simulink model "simulation"  (R2020a)
settings: Solver=ode4  StartTime=0.0  StopTime=10.0  FixedStep=dt  RelTol=1e-3
values from neighbouring files (symbols this model uses):
  alt0 = 600    [initializeSim.m]
  dt = 0.1    [dryden_wind_model.m]    (also in filters.m; full_sim_and_filter_loop.m = 0.01; getDynamicsJacobian.m; initializeSim.m = 0.01)
  F = [0;0;0]    [simple_sim.m]
  initCovarianceEkf = diag([1e-3, 1e-3,                            2, 5e-3,                            1e-4, 1e-4,                            10, 10])    [initializeSim.m]
  initEstimateEkf = [0, 0,                     initGroundSpeedEst, initAttitude(3),                     windNorthStatic + 4*randn, windEastStatic + 4*randn,                     0, 0]    [initializeSim.m]
  q = uKF(2)    [dynJacobian.m]    (also in getDynamicsJacobian.m; getDynamicsJacobianTest.m; getStateTransitionDynamics.m; simple_sim.m)
  Qekf = diag([1e-5, 1e-5,               1, 1e-3,               1, 1,               1, 1])    [initializeSim.m]
  r = uKF(3)    [dynJacobian.m]    (also in getDynamicsJacobian.m; getDynamicsJacobianTest.m; getStateTransitionDynamics.m; simple_sim.m)
  Rekf = diag([1, 1,               1, 1e-3,               1, 1])    [initializeSim.m]
  sensorNoiseFlag = 1    [initializeSim.m]
  staticWindFlag = 1    [initializeSim.m]
  turbulentWindFlag = 1    [initializeSim.m]
  windDownStatic = 0    [initializeSim.m]
  windEastStatic = -9    [initializeSim.m]
  windNorthStatic = 14    [initializeSim.m]
undefined symbols (not defined in the file or in its folder): Light, MIL
libraries: shared6dof x1, aerolibwind2 x1
settings Model: Creator=Don  LastModifiedBy=don

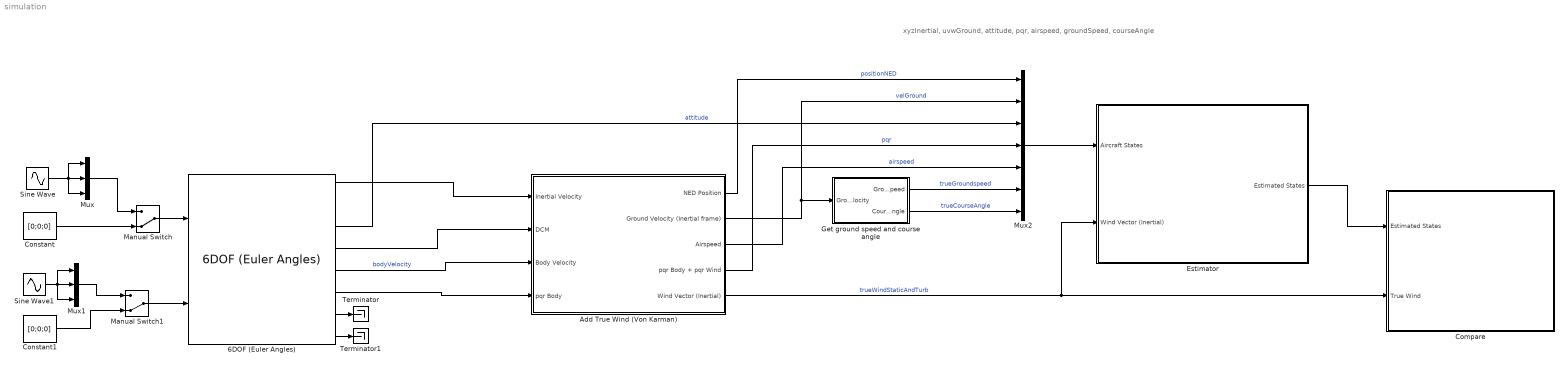
== system simulation ==
  note: xyzInertial, uvwGround, attitude, pqr, airspeed, groundSpeed, courseAngle
  6DOF (Euler Angles) : shared6dof/6DOF (Euler Angles)  units=Metric (MKS)  mtype=Fixed  rep=Euler Angles  xme_0=[0 0 -abs(alt0)]  Vm_0=initVelBody  eul_0=initAttitude  pm_0=[0 0 0]  mass_0=mass  mass_e=0.5  mass_f=2.0  inertia=J  inertia_e=eye(3)  inertia_f=2*eye(3)  k_quat=1.0  vre_flag=on  abi_flag=off  aMode=0  xme_statename=''  Vm_statename=''  eul_statename=''  quat_statename=''  pm_statename=''  mass_statename=''
      settings: SourceProductBaseCode=AE,PW,MT,VE,VP
  Add True Wind (Von Karman) : Subsystem
  Compare : Subsystem
  Constant : Constant  Value=[0;0;0]
  Constant1 : Constant  Value=[0;0;0]
  Estimator : Subsystem
  Get ground speed and course angle : Subsystem
  Manual Switch : ManualSwitch  CurrentSetting=0
  Manual Switch1 : ManualSwitch  CurrentSetting=0
  Mux : Mux  Inputs=3
  Mux1 : Mux  Inputs=3
  Mux2 : Mux  Inputs=7
  Sine Wave : Sin  SampleTime=0
  Sine Wave1 : Sin  SampleTime=0
  Terminator : Terminator
  Terminator1 : Terminator
  wires:
  Constant/1 -> Manual Switch/2
  Constant1/1 -> Manual Switch1/2
  6DOF (Euler Angles)/1 -> Add True Wind (Von Karman)/1(Inertial Velocity)
  6DOF (Euler Angles)/4 -> Add True Wind (Von Karman)/2(DCM)
  6DOF (Euler Angles)/5 -> Add True Wind (Von Karman)/3(Body Velocity)  "bodyVelocity"
  6DOF (Euler Angles)/6 -> Add True Wind (Von Karman)/4(pqr Body)
  Manual Switch/1 -> 6DOF (Euler Angles)/1
  Manual Switch1/1 -> 6DOF (Euler Angles)/2
  Sine Wave/1 -> Mux/2, Mux/1, Mux/3
  Mux/1 -> Manual Switch/1
  Sine Wave1/1 -> Mux1/2, Mux1/1, Mux1/3
  Mux1/1 -> Manual Switch1/1
  Add True Wind (Von Karman)/2(Ground Velocity (Inertial frame)) -> Mux2/2, Get ground speed and course angle/1(Ground Velocity)  "velGround"
  6DOF (Euler Angles)/3 -> Mux2/3  "attitude"
  Mux2/1 -> Estimator/1(Aircraft States)
  Add True Wind (Von Karman)/3(Airspeed) -> Mux2/5  "airspeed"
  6DOF (Euler Angles)/7 -> Terminator/1
  6DOF (Euler Angles)/8 -> Terminator1/1
  Estimator/1(Estimated States) -> Compare/1(Estimated States)
  Add True Wind (Von Karman)/4(pqr Body + pqr Wind) -> Mux2/4  "pqr"
  Get ground speed and course angle/1(Ground Speed) -> Mux2/6  "trueGroundspeed"
  Add True Wind (Von Karman)/1(NED Position) -> Mux2/1  "positionNED"
  Add True Wind (Von Karman)/5(Wind Vector (Inertial)) -> Compare/2(True Wind), Estimator/2(Wind Vector (Inertial))  "trueWindStaticAndTurb"
  Get ground speed and course angle/2(Course Angle) -> Mux2/7  "trueCourseAngle"

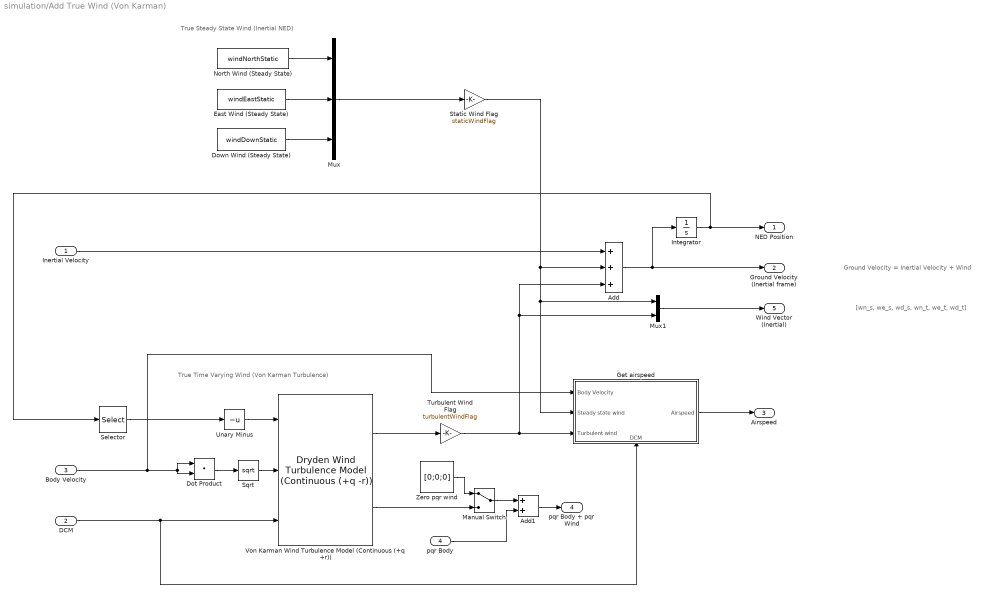
== system simulation/Add True Wind (Von Karman) ==
  note: [wn_s, we_s, wd_s, wn_t, we_t, wd_t]
  note: Ground Velocity = Inertial Velocity + Wind
  note: True Time Varying Wind (Von Karman Turbulence)
  note: True Steady State Wind (Inertial NED)
  Inertial Velocity : Inport
  DCM : Inport  Port=2
  Body Velocity : Inport  Port=3
  pqr Body : Inport  Port=4
  Add : Sum  Inputs=+++
  Add1 : Sum
  Dot Product : DotProduct  InputSameDT=on  OutDataTypeStr=Inherit: Inherit via internal rule
  Down Wind (Steady State) : Constant  Value=windDownStatic
  East Wind (Steady State) : Constant  Value=windEastStatic
  Get airspeed : Subsystem
      settings: PortSchema="{\"entries\":[{\"content\":{\"sides\":[{\"content\":{\"connectorIds\":[\"In1\",\"In2\",\"In3\"]},\"type\":\"ConnectorPlacement.EquallySpacedRectSide\",\"uuid\":\"813c2b5b-04f3-4ec3-a969-2504c20ca38b\"},{\"content\":{\"connectorIds\":[\"Out1\"],\"side\":\"RIGHT\"},\"type\":\"ConnectorPlacement.EquallySpacedRectSide\",\"uuid\":\"9f878792-4dd4-4000-acee-7f28349bdd5f\"},{\"content\":{\"connectorIds\":[],\"side\":\"TOP\"},\"type\":\"ConnectorPlacement.EquallySpacedRectSide\",\"uuid\":\"3d2ef613-18a7-4015-9ddb-8a03be605fb8\"},{\"content\":{\"connectorIds\":[\"In4\"],\"side\":\"BOTTOM\"},\"type\":\"ConnectorPlacement.EquallySpacedRectSide\",\"uuid\":\"121bcea6-4847-4a17-8a68-e62f0e126d50\"}]},\"type\":\"ConnectorPlacement.EquallySpacedConnector\",\"uuid\":\"0bfc4666-1d36-45c8-946f-537367ff2a54\"}],\"packageUris\":[\"http://schema.mathworks.com/mf0/Connector/19700101\"],\"version\":\"1.0\"}"
  Integrator : Integrator  InitialCondition=[0, 0, -abs(alt0)]
  Manual Switch : ManualSwitch
  Mux : Mux  Inputs=3
  Mux1 : Mux  Inputs=2
  North Wind (Steady State) : Constant  Value=windNorthStatic
  Selector : Selector  InputPortWidth=3  IndexOptions=Index vector (dialog)  Indices=3  OutputSizes=1
  Sqrt : Sqrt  SaturateOnIntegerOverflow=on
  Static Wind Flag : Gain  Gain=staticWindFlag
  Turbulent Wind Flag : Gain  Gain=turbulentWindFlag
  Unary Minus : UnaryMinus
  Von Karman Wind Turbulence Model (Continuous (+q +r)) : aerolibwind2/Dryden Wind Turbulence Model  (Continuous (+q -r))  units=Metric (MKS)  spec=MIL-F-8785C  model=Continuous Von Karman (+q +r)  W20=15  Wdeg=0  TurbProb=10^-2 - Light  L_high=762  Wingspan=10  ts=0.1  Seed=[23341 23342 23343 23344]  T_on=on
  Zero pqr wind : Constant  Value=[0;0;0]
  NED Position : Outport  PortDimensions=3
  Ground Velocity (Inertial frame) : Outport  Port=2
  Airspeed : Outport  Port=3  PortDimensions=1
  pqr Body + pqr Wind : Outport  Port=4
  Wind Vector (Inertial) : Outport  Port=5
  wires:
  Sqrt/1 -> Von Karman Wind Turbulence Model (Continuous (+q +r))/2
  Selector/1 -> Unary Minus/1
  Von Karman Wind Turbulence Model (Continuous (+q +r))/1 -> Turbulent Wind Flag/1
  Unary Minus/1 -> Von Karman Wind Turbulence Model (Continuous (+q +r))/1
  DCM/1 -> Get airspeed/4(DCM), Von Karman Wind Turbulence Model (Continuous (+q +r))/3
  Body Velocity/1 -> Get airspeed/1(Body Velocity), Dot Product/2, Dot Product/1
  Von Karman Wind Turbulence Model (Continuous (+q +r))/2 -> Manual Switch/2
  Add/1 -> Ground Velocity (Inertial frame)/1, Integrator/1
  Add1/1 -> pqr Body + pqr Wind/1
  Inertial Velocity/1 -> Add/1
  pqr Body/1 -> Add1/2
  North Wind (Steady State)/1 -> Mux/1
  East Wind (Steady State)/1 -> Mux/2
  Down Wind (Steady State)/1 -> Mux/3
  Mux/1 -> Static Wind Flag/1
  Manual Switch/1 -> Add1/1
  Zero pqr wind/1 -> Manual Switch/1
  Get airspeed/1(Airspeed) -> Airspeed/1
  Dot Product/1 -> Sqrt/1
  Mux1/1 -> Wind Vector (Inertial)/1
  Integrator/1 -> Selector/1, NED Position/1
  Turbulent Wind Flag/1 -> Get airspeed/3(Turbulent wind), Add/3, Mux1/2
  Static Wind Flag/1 -> Mux1/1, Get airspeed/2(Steady state wind), Add/2

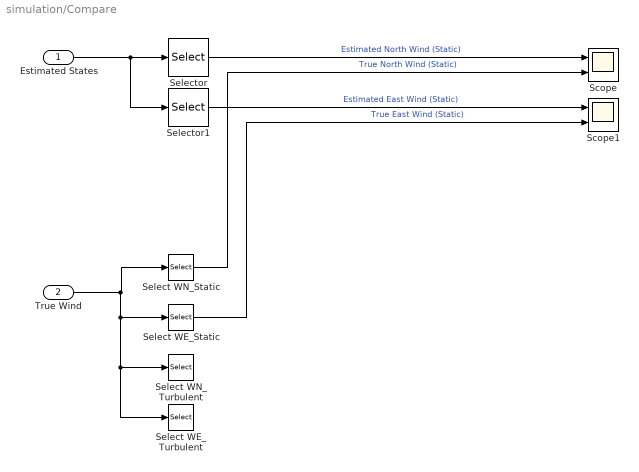
== system simulation/Compare ==
  Estimated States : Inport
  True Wind : Inport  Port=2
  Scope : Scope  NumInputPorts=2
  Scope1 : Scope  NumInputPorts=2
  Select WE_Static : Selector  InputPortWidth=6  IndexOptions=Index vector (dialog)  Indices=2  OutputSizes=1
  Select WE_Turbulent : Selector  InputPortWidth=6  IndexOptions=Index vector (dialog)  Indices=5  OutputSizes=1
  Select WN_Static : Selector  InputPortWidth=6  IndexOptions=Index vector (dialog)  Indices=1  OutputSizes=1
  Select WN_Turbulent : Selector  InputPortWidth=6  IndexOptions=Index vector (dialog)  Indices=4  OutputSizes=1
  Selector : Selector  InputPortWidth=6  IndexOptions=Index vector (dialog)  Indices=5  OutputSizes=1
  Selector1 : Selector  InputPortWidth=6  IndexOptions=Index vector (dialog)  Indices=6  OutputSizes=1
  wires:
  Estimated States/1 -> Selector1/1, Selector/1
  True Wind/1 -> Select WE_Turbulent/1, Select WN_Turbulent/1, Select WE_Static/1, Select WN_Static/1
  Selector/1 -> Scope/1  "Estimated North Wind (Static)"
  Select WN_Static/1 -> Scope/2  "True North Wind (Static)"
  Selector1/1 -> Scope1/1  "Estimated East Wind (Static)"
  Select WE_Static/1 -> Scope1/2  "True East Wind (Static)"

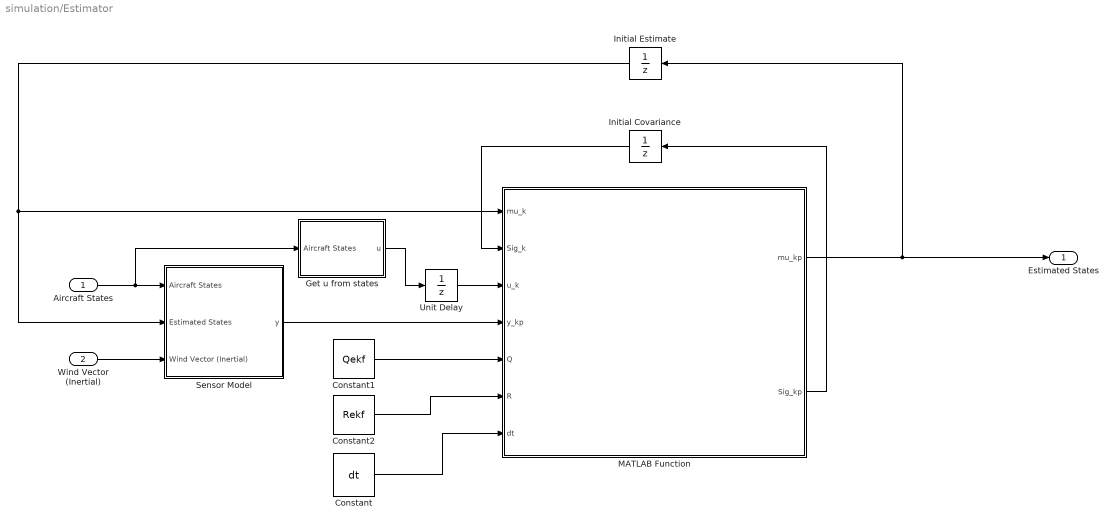
== system simulation/Estimator ==
  Aircraft States : Inport
  Wind Vector (Inertial) : Inport  Port=2
  Constant : Constant  Value=dt
  Constant1 : Constant  Value=Qekf
  Constant2 : Constant  Value=Rekf
  Get u from states : Subsystem
  Initial Covariance : UnitDelay  InitialCondition=initCovarianceEkf  SampleTime=-1  HasFrameUpgradeWarning=on
  Initial Estimate : UnitDelay  InitialCondition=initEstimateEkf  SampleTime=-1  HasFrameUpgradeWarning=on
  MATLAB Function : MATLAB Function  TreatAsAtomicUnit=on
  Sensor Model : Subsystem
  Unit Delay : UnitDelay  SampleTime=-1  HasFrameUpgradeWarning=on
  Estimated States : Outport
  wires:
  Constant/1 -> MATLAB Function/7(dt)
  Aircraft States/1 -> Get u from states/1(Aircraft States), Sensor Model/1(Aircraft States)
  Sensor Model/1(y) -> MATLAB Function/4(y_kp)
  MATLAB Function/1(mu_kp) -> Initial Estimate/1, Estimated States/1
  Constant1/1 -> MATLAB Function/5(Q)
  Constant2/1 -> MATLAB Function/6(R)
  Initial Estimate/1 -> MATLAB Function/1(mu_k), Sensor Model/2(Estimated States)
  MATLAB Function/2(Sig_kp) -> Initial Covariance/1
  Initial Covariance/1 -> MATLAB Function/2(Sig_k)
  Get u from states/1(u) -> Unit Delay/1
  Wind Vector (Inertial)/1 -> Sensor Model/3(Wind Vector (Inertial))
  Unit Delay/1 -> MATLAB Function/3(u_k)

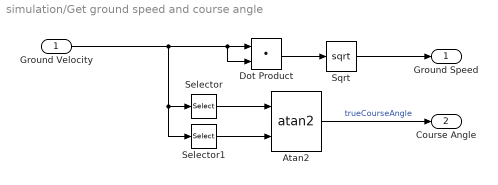
== system simulation/Get ground speed and course angle ==
  Ground Velocity : Inport
  Atan2 : Trigonometry  Operator=atan2
  Dot Product : DotProduct  InputSameDT=on  OutDataTypeStr=Inherit: Inherit via internal rule
  Selector : Selector  InputPortWidth=3  IndexOptions=Index vector (dialog)  Indices=2  OutputSizes=1
  Selector1 : Selector  InputPortWidth=3  IndexOptions=Index vector (dialog)  Indices=1  OutputSizes=1
  Sqrt : Sqrt  SaturateOnIntegerOverflow=on
  Ground Speed : Outport
  Course Angle : Outport  Port=2
  wires:
  Selector1/1 -> Atan2/2
  Selector/1 -> Atan2/1
  Ground Velocity/1 -> Dot Product/2, Dot Product/1, Selector1/1, Selector/1
  Atan2/1 -> Course Angle/1  "trueCourseAngle"
  Dot Product/1 -> Sqrt/1
  Sqrt/1 -> Ground Speed/1

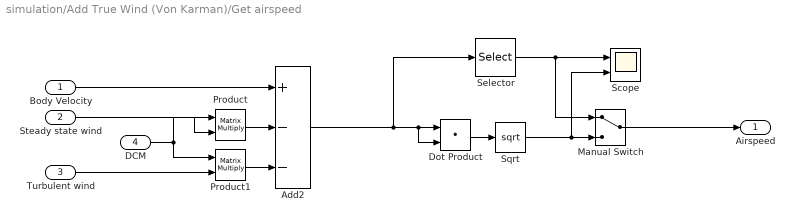
== system simulation/Add True Wind (Von Karman)/Get airspeed ==
  Body Velocity : Inport
  Steady state wind : Inport  Port=2
  Turbulent wind : Inport  Port=3
  DCM : Inport  Port=4
  Add2 : Sum  Inputs=+--
  Dot Product : DotProduct  InputSameDT=on  OutDataTypeStr=Inherit: Inherit via internal rule
  Manual Switch : ManualSwitch
  Product : Product  Multiplication=Matrix(*)
  Product1 : Product  Multiplication=Matrix(*)
  Scope : Scope  NumInputPorts=2
  Selector : Selector  InputPortWidth=3  IndexOptions=Index vector (dialog)  Indices=1  OutputSizes=1
  Sqrt : Sqrt  SaturateOnIntegerOverflow=on
  Airspeed : Outport
  wires:
  Body Velocity/1 -> Add2/1
  Steady state wind/1 -> Product/2
  Add2/1 -> Dot Product/2, Dot Product/1, Selector/1
  Turbulent wind/1 -> Product1/2
  DCM/1 -> Product/1, Product1/1
  Product/1 -> Add2/2
  Product1/1 -> Add2/3
  Manual Switch/1 -> Airspeed/1
  Selector/1 -> Manual Switch/1, Scope/1
  Dot Product/1 -> Sqrt/1
  Sqrt/1 -> Scope/2, Manual Switch/2

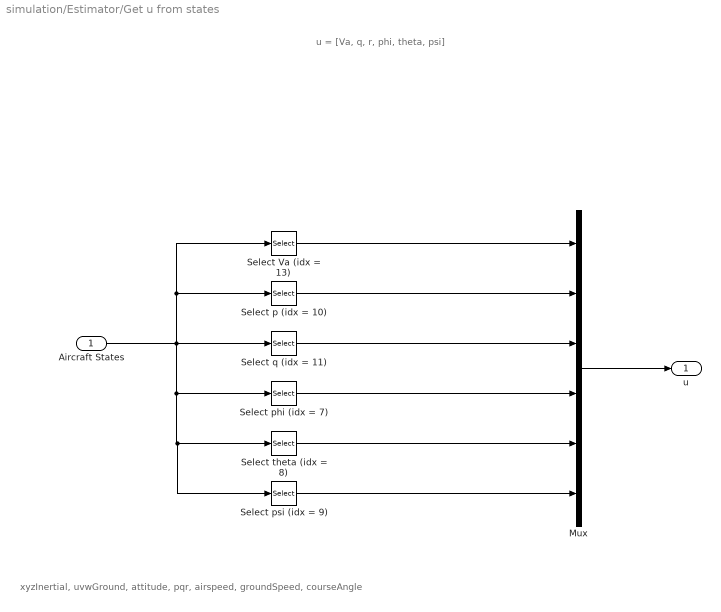
== system simulation/Estimator/Get u from states ==
  note: u = [Va, q, r, phi, theta, psi]
  note: xyzInertial, uvwGround, attitude, pqr, airspeed, groundSpeed, courseAngle
  Aircraft States : Inport
  Mux : Mux  Inputs=6
  Select Va (idx = 13) : Selector  InputPortWidth=15  IndexOptions=Index vector (dialog)  Indices=13  OutputSizes=1
  Select p (idx = 10) : Selector  InputPortWidth=15  IndexOptions=Index vector (dialog)  Indices=10  OutputSizes=1
  Select phi (idx = 7) : Selector  InputPortWidth=15  IndexOptions=Index vector (dialog)  Indices=7  OutputSizes=1
  Select psi (idx = 9) : Selector  InputPortWidth=15  IndexOptions=Index vector (dialog)  Indices=9  OutputSizes=1
  Select q (idx = 11) : Selector  InputPortWidth=15  IndexOptions=Index vector (dialog)  Indices=11  OutputSizes=1
  Select theta (idx = 8) : Selector  InputPortWidth=15  IndexOptions=Index vector (dialog)  Indices=8  OutputSizes=1
  u : Outport
  wires:
  Aircraft States/1 -> Select psi (idx = 9)/1, Select theta (idx = 8)/1, Select phi (idx = 7)/1, Select q (idx = 11)/1, Select p (idx = 10)/1, Select Va (idx = 13)/1
  Mux/1 -> u/1
  Select p (idx = 10)/1 -> Mux/2
  Select Va (idx = 13)/1 -> Mux/1
  Select q (idx = 11)/1 -> Mux/3
  Select phi (idx = 7)/1 -> Mux/4
  Select theta (idx = 8)/1 -> Mux/5
  Select psi (idx = 9)/1 -> Mux/6

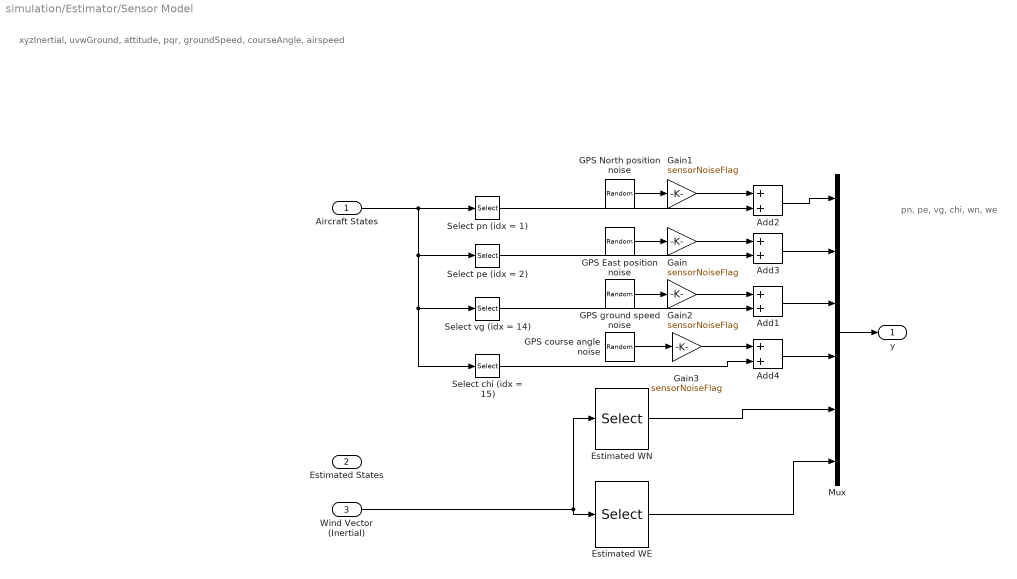
== system simulation/Estimator/Sensor Model ==
  note: pn, pe, vg, chi, wn, we
  note: xyzInertial, uvwGround, attitude, pqr, groundSpeed, courseAngle, airspeed
  Aircraft States : Inport
  Estimated States : Inport  Port=2
  Wind Vector (Inertial) : Inport  Port=3
  Add{1..4} (4 alike) : Sum
  Estimated WE : Selector  InputPortWidth=6  IndexOptions=Index vector (dialog)  Indices=6  OutputSizes=1
  Estimated WN : Selector  InputPortWidth=6  IndexOptions=Index vector (dialog)  Indices=5  OutputSizes=1
  GPS East position noise : RandomNumber  SampleTime=0.1
  GPS North position noise : RandomNumber  SampleTime=0.1
  GPS course angle noise : RandomNumber  SampleTime=0.1
  GPS ground speed noise : RandomNumber  SampleTime=0.1
  Gain{,1..3} (4 alike) : Gain  Gain=sensorNoiseFlag
  Mux : Mux  Inputs=6
  Select chi (idx = 15) : Selector  InputPortWidth=15  IndexOptions=Index vector (dialog)  Indices=15  OutputSizes=1
  Select pe (idx = 2) : Selector  InputPortWidth=15  IndexOptions=Index vector (dialog)  Indices=2  OutputSizes=1
  Select pn (idx = 1) : Selector  InputPortWidth=15  IndexOptions=Index vector (dialog)  Indices=1  OutputSizes=1
  Select vg (idx = 14) : Selector  InputPortWidth=15  IndexOptions=Index vector (dialog)  Indices=14  OutputSizes=1
  y : Outport
  wires:
  Aircraft States/1 -> Select chi (idx = 15)/1, Select vg (idx = 14)/1, Select pe (idx = 2)/1, Select pn (idx = 1)/1
  Mux/1 -> y/1
  GPS ground speed noise/1 -> Gain2/1
  Add2/1 -> Mux/1
  Select pn (idx = 1)/1 -> Add2/2
  GPS North position noise/1 -> Gain1/1
  Add3/1 -> Mux/2
  GPS East position noise/1 -> Gain/1
  Select pe (idx = 2)/1 -> Add3/2
  GPS course angle noise/1 -> Gain3/1
  Add4/1 -> Mux/4
  Add1/1 -> Mux/3
  Wind Vector (Inertial)/1 -> Estimated WN/1, Estimated WE/1
  Estimated WN/1 -> Mux/5
  Estimated WE/1 -> Mux/6
  Gain/1 -> Add3/1
  Gain1/1 -> Add2/1
  Gain2/1 -> Add1/1
  Gain3/1 -> Add4/1
  Select vg (idx = 14)/1 -> Add1/2
  Select chi (idx = 15)/1 -> Add4/2

== matlab function simulation/Estimator/MATLAB Function ==
  data: mu_k input; mu_kp output; Sig_k input; u_k input; y_kp input; Q input; R input; dt input; Sig_kp output
function [mu_kp, Sig_kp] = extendedKalmanFilter(mu_k, Sig_k, u_k, y_kp, Q, R, dt)
    % Prediction step
    A = getDynamicsJacobian(mu_k, u_k);
    mu_pred = dynamics(mu_k, u_k, dt);
    Sig_pred = A*Sig_k*A' + Q;

    % Update step
    C = getMeasurementJacobian(mu_pred);
    ybar = y_kp - getMeasurementModel(mu_pred, u_k);
    K = Sig_pred*C'/(C*Sig_pred*C' + R); % Kalman gain
    mu_kp = mu_pred + K*ybar;
    Sig_kp = Sig_pred - K*C*Sig_pred;
end
